simulink model "model_1a"  (R2019b)
settings: Solver=VariableStepAuto  StartTime=0.0  StopTime=simulation_time  RelTol=1e-3
values from neighbouring files (symbols this model uses):
  deltat = sample_time    (= 0.004)    [params.m]
  Gs = tf(K, [tau 1])    [params.m]
  Kc = pi.Kc    [params.m]
  sample_time = 1/5*wn    (= 0.004)    [params.m]
  step_amplitude = 67    [params.m]
  tauI = pi.tauI    [params.m]
  Umax = 1    [params.m]
  Umin = 0    [params.m]
settings Model: Creator=adityaaaap  LastModifiedBy=adityaaaap

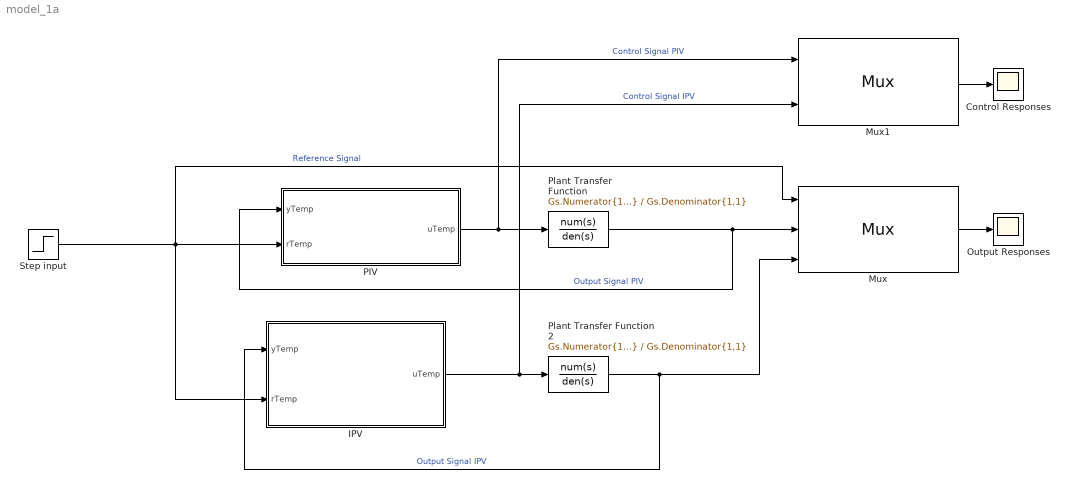
== system model_1a ==
  Control Responses : Scope
  "IPV " : MATLAB Function  TreatAsAtomicUnit=on
  Mux : Mux  Inputs=3
      settings: DisplayOption=signals
  Mux1 : Mux  Inputs=2
      settings: DisplayOption=signals
  Output Responses : Scope
  "PIV " : MATLAB Function  TreatAsAtomicUnit=on
  Plant Transfer Function : TransferFcn  Numerator=Gs.Numerator{1,1}  Denominator=Gs.Denominator{1,1}
  Plant Transfer Function 2 : TransferFcn  Numerator=Gs.Numerator{1,1}  Denominator=Gs.Denominator{1,1}
  Step input : Step  Time=0  After=step_amplitude  SampleTime=sample_time
  wires:
  Step input/1 -> Mux/1, "IPV "/2(rTemp), "PIV "/2(rTemp)  "Reference Signal"
  "PIV "/1(uTemp) -> Plant Transfer Function/1, Mux1/1  "Control Signal PIV"
  Plant Transfer Function/1 -> "PIV "/1(yTemp), Mux/2  "Output Signal PIV"
  Mux/1 -> Output Responses/1
  "IPV "/1(uTemp) -> Mux1/2, Plant Transfer Function 2/1  "Control Signal IPV"
  Plant Transfer Function 2/1 -> Mux/3, "IPV "/1(yTemp)  "Output Signal IPV"
  Mux1/1 -> Control Responses/1

== matlab function model_1a/IPV  ==
  settings: updateMethod=DISCRETE  sampleTime=deltat
  data: yTemp input; uTemp output; rTemp input; Kc parameter; tauI parameter; deltat parameter; Umin parameter; Umax parameter
function uTemp = IPV(yTemp,rTemp,Kc, tauI, deltat, Umin, Umax)
    persistent uPast 
    if isempty(uPast)
        uPast=0;
    end
    
    persistent yPast 
    if isempty(yPast)
        yPast=0; 
    end
    
    persistent uDPast 
    if isempty(uDPast)
        uDPast=0;
    end
    
    persistent rPast 
    if isempty(rPast)
        rPast=0;
    end
   
    uTemp = uPast+...
        Kc*(-yTemp+yPast)+ ...
        (Kc*deltat)/tauI*(rTemp-yTemp);

    if (uTemp>Umax) 
        uTemp=Umax;
    end
    
    if (uTemp<Umin) 
        uTemp=Umin; 
    end
    
    uPast=uTemp; 
    yPast=yTemp; 
    rPast=rTemp;
end

== matlab function model_1a/PIV  ==
  settings: updateMethod=DISCRETE  sampleTime=deltat
  data: yTemp input; uTemp output; rTemp input; Kc parameter; tauI parameter; deltat parameter; Umin parameter; Umax parameter
function uTemp = PIV(yTemp,rTemp,Kc, tauI, deltat, Umin, Umax)
    persistent uPast 
    if isempty(uPast)
        uPast=0;
    end
    
    persistent yPast 
    if isempty(yPast)
        yPast=0; 
    end
    
    persistent uDPast 
    if isempty(uDPast)
        uDPast=0;
    end
    
    persistent rPast 
    if isempty(rPast)
        rPast=0;
    end
    
    
    uTemp=uPast + ...
        Kc*(rTemp-yTemp-rPast+yPast) + ...
        ((Kc*deltat)/tauI)*(rTemp-yTemp);
    

    if (uTemp>Umax) 
        uTemp=Umax;
    end
    
    if (uTemp<Umin) 
        uTemp=Umin; 
    end
    
    uPast=uTemp; 
    yPast=yTemp; 
    rPast=rTemp;
end
